simulink model "up_counter_2bit"  (R2025b)
settings: Solver=VariableStepAuto  StartTime=0.0  StopTime=10.0  RelTol=1e-3
libraries: simulink_extras x3
settings Model: Creator=Johan  LastModifiedBy=Johan

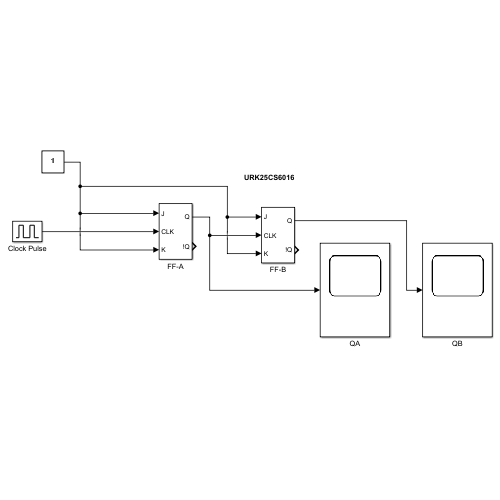
[thumbnail: Simulink's stored preview of the top-level diagram]
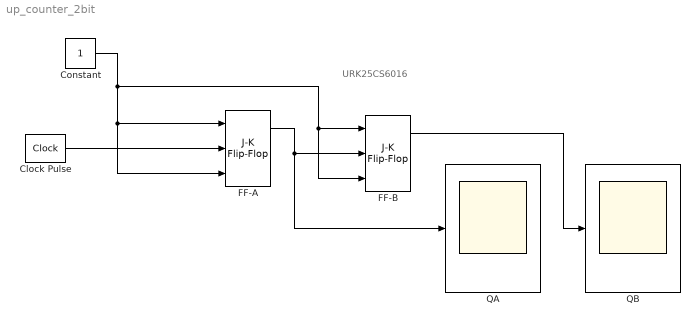
== system up_counter_2bit ==
  note: URK25CS6016
  Clock Pulse : simulink_extras/Flip Flops/Clock  period=2
  Constant : Constant  OutDataTypeStr=boolean
  FF-A : simulink_extras/Flip Flops/J-K Flip-Flop  initial_condition=0
  FF-B : simulink_extras/Flip Flops/J-K Flip-Flop  initial_condition=0
  QA : Scope
      settings: ActiveDisplayYMinimum=-0.16613828502415451  ActiveDisplayYMaximum=1.1463617149758454
  QB : Scope
      settings: ActiveDisplayYMinimum=-0.12499999999999997  ActiveDisplayYMaximum=1.125
  wires:
  Constant/1 -> FF-A/3, FF-A/1, FF-B/3, FF-B/1
  Clock Pulse/1 -> FF-A/2
  FF-A/1 -> QA/1, FF-B/2
  FF-B/1 -> QB/1
